simulink model "WFXXPIDb"  (Simulink 5.0)
settings: Solver=ode4  StartTime=0.0  StopTime=8000  FixedStep=20  RelTol=1e-3
settings Model: LastModifiedBy=ThinkPad

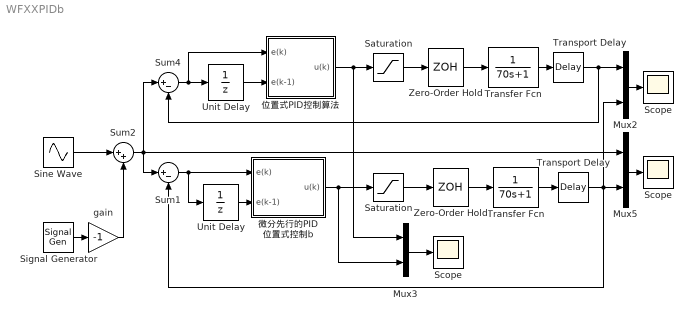
== system WFXXPIDb ==
  " Scope  " : Scope
      settings: YMin=-1.5  YMax=1.5  SaveName=WFXXPIDbu  DataFormat=Array  MaxDataPoints=500000
  Mux2 : Mux  Inputs=2
  Mux3 : Mux  Inputs=2
  Mux5 : Mux  Inputs=2
  Saturation : Saturate  UpperLimit=10  LowerLimit=-10
  "Saturation " : Saturate  UpperLimit=10  LowerLimit=-10
  Scope : Scope
      settings: YMin=-1.5  YMax=1.5  SaveName=WFXXPIDPIDby  DataFormat=Array  MaxDataPoints=500000
  "Scope " : Scope
      settings: YMin=-1.5  YMax=1.5  SaveName=WFXXPIDbry  DataFormat=Array  MaxDataPoints=500000
  "Signal Generator " : SignalGenerator  WaveForm=square  Frequency=0.0005*pi  Units=rad/sec
  "Sine Wave " : Sin  Amplitude=0.05  Frequency=0.03*pi  SampleTime=0
  Sum1 : Sum  Inputs=|+-  SaturateOnIntegerOverflow=on
  Sum2 : Sum  Inputs=|++  SaturateOnIntegerOverflow=on
  Sum4 : Sum  Inputs=|+-  SaturateOnIntegerOverflow=on
  Transfer Fcn : TransferFcn  Denominator=[70 1]
  "Transfer Fcn " : TransferFcn  Denominator=[70 1]
  Transport Delay : TransportDelay  DelayTime=80
  "Transport Delay " : TransportDelay  DelayTime=80
  Unit Delay : UnitDelay  SampleTime=20
  "Unit Delay " : UnitDelay  SampleTime=20
  Zero-Order Hold : ZeroOrderHold  SampleTime=20
  "Zero-Order Hold " : ZeroOrderHold  SampleTime=20
  gain : Gain  Gain=-1  SaturateOnIntegerOverflow=on
  微分先行的PID 位置式控制b : Subsystem
  "位置式PID控制算法 " : Subsystem
  wires:
  Sum2/1 -> Sum4/1, Mux5/1, Sum1/1
  Transfer Fcn/1 -> Transport Delay/1
  微分先行的PID 位置式控制b/1(u(k)) -> Saturation/1, Mux3/2
  Zero-Order Hold/1 -> Transfer Fcn/1
  Mux5/1 -> "Scope "/1
  Transport Delay/1 -> Mux5/2, Mux2/2, Sum1/2
  "Transfer Fcn "/1 -> "Transport Delay "/1
  "位置式PID控制算法 "/1(u(k)) -> "Saturation "/1, Mux3/1
  Sum4/1 -> "Unit Delay "/1, "位置式PID控制算法 "/1(e(k))
  "Zero-Order Hold "/1 -> "Transfer Fcn "/1
  Mux2/1 -> Scope/1
  "Transport Delay "/1 -> Mux2/1, Sum4/2
  "Unit Delay "/1 -> "位置式PID控制算法 "/2(e(k-1))
  Unit Delay/1 -> 微分先行的PID 位置式控制b/2(e(k-1))
  "Sine Wave "/1 -> Sum2/1
  "Signal Generator "/1 -> gain/1
  gain/1 -> Sum2/2
  Saturation/1 -> Zero-Order Hold/1
  "Saturation "/1 -> "Zero-Order Hold "/1
  Mux3/1 -> " Scope  "/1
  Sum1/1 -> 微分先行的PID 位置式控制b/1(e(k)), Unit Delay/1

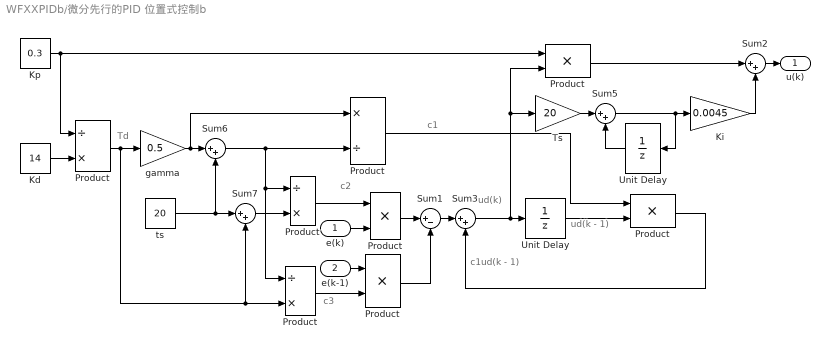
== system WFXXPIDb/微分先行的PID 位置式控制b ==
  note: c1ud(k－1)
  note: Td
  note: c2
  note: c3
  note: c1
  note: ud(k－1)
  note: ud(k)
  e(k) : Inport
  e(k-1) : Inport  Port=2
  " Product " : Product  SaturateOnIntegerOverflow=on
  " Product  " : Product  Inputs=/*  SaturateOnIntegerOverflow=on
  " Product   " : Product  Inputs=/*  SaturateOnIntegerOverflow=on
  " Product    " : Product  SaturateOnIntegerOverflow=on
  " Product     " : Product  SaturateOnIntegerOverflow=on
  Kd : Constant  Value=14
  Ki : Gain  Gain=0.0045  SaturateOnIntegerOverflow=on
  Kp : Constant  Value=0.3
  Product : Product  SaturateOnIntegerOverflow=on
  "Product " : Product  Inputs=/*  SaturateOnIntegerOverflow=on
  "Product   " : Product  Inputs=*/  SaturateOnIntegerOverflow=on
  Sum1 : Sum  Inputs=|+-  SaturateOnIntegerOverflow=on
  Sum{2..3,5..7} (5 alike) : Sum  Inputs=|++  SaturateOnIntegerOverflow=on
  Ts : Gain  Gain=20  SaturateOnIntegerOverflow=on
  Unit Delay : UnitDelay  Orientation=left  SampleTime=20
  "Unit Delay " : UnitDelay  SampleTime=20
  gamma : Gain  Gain=0.5  SaturateOnIntegerOverflow=on
  ts : Constant  Value=20
  u(k) : Outport
  wires:
  Ts/1 -> Sum5/1
  Sum5/1 -> Unit Delay/1, Ki/1
  Unit Delay/1 -> Sum5/2
  Ki/1 -> Sum2/2
  Sum1/1 -> Sum3/1
  Sum2/1 -> u(k)/1
  Sum3/1 -> "Unit Delay "/1, Product/2, Ts/1
  Kp/1 -> Product/1, "Product "/1
  Kd/1 -> "Product "/2
  ts/1 -> Sum6/2, Sum7/1
  Sum6/1 -> "Product   "/2, " Product  "/1, " Product   "/1
  "Product "/1 -> Sum7/2, " Product   "/2, gamma/1
  Sum7/1 -> " Product  "/2
  " Product  "/1 -> " Product     "/1
  " Product   "/1 -> " Product    "/2
  e(k)/1 -> " Product     "/2
  " Product     "/1 -> Sum1/1
  e(k-1)/1 -> " Product    "/1
  " Product    "/1 -> Sum1/2
  "Product   "/1 -> " Product "/1
  " Product "/1 -> Sum3/2
  "Unit Delay "/1 -> " Product "/2
  gamma/1 -> Sum6/1, "Product   "/1
  Product/1 -> Sum2/1

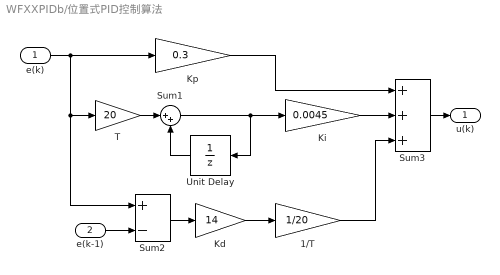
== system WFXXPIDb/位置式PID控制算法  ==
  e(k) : Inport
  e(k-1) : Inport  Port=2
  1/T : Gain  Gain=1/20  SaturateOnIntegerOverflow=on
  Kd : Gain  Gain=14  SaturateOnIntegerOverflow=on
  Ki : Gain  Gain=0.0045  SaturateOnIntegerOverflow=on
  Kp : Gain  Gain=0.3  SaturateOnIntegerOverflow=on
  Sum1 : Sum  Inputs=|++  SaturateOnIntegerOverflow=on
  Sum2 : Sum  Inputs=+-  SaturateOnIntegerOverflow=on
  Sum3 : Sum  Inputs=+++  SaturateOnIntegerOverflow=on
  T : Gain  Gain=20  SaturateOnIntegerOverflow=on
  Unit Delay : UnitDelay  Orientation=left  SampleTime=20
  u(k) : Outport
  wires:
  Sum2/1 -> Kd/1
  e(k)/1 -> Kp/1, Sum2/1, T/1
  Kp/1 -> Sum3/1
  Ki/1 -> Sum3/2
  Sum3/1 -> u(k)/1
  Kd/1 -> 1/T/1
  e(k-1)/1 -> Sum2/2
  1/T/1 -> Sum3/3
  Sum1/1 -> Unit Delay/1, Ki/1
  Unit Delay/1 -> Sum1/2
  T/1 -> Sum1/1
